simulink model "MenakaModel"  (R2022a)
settings: Solver=ode23tb  StartTime=0.0  StopTime=4  MaxStep=10/(60*24)  RelTol=1e-3
model workspace (MAT data in the model file):
  clima__A_c = 3295.16408265
  clima__A_f = 3100.53942116
  clima__G0 = [0.05; 0.00070738]
  clima__H = 7.9995824611
  clima__T0 = [287.15; 287.15; 287.15; 287.15]
  clima__T_ss = 280.150340169
  clima__alpha_c = 0.0100640347387
  clima__alpha_f = 0.0111385012129
  clima__alpha_i = 0.1
  clima__c_s = [1081 1081]
  clima__cd_c = 8736
  clima__d_c = 1.5
  clima__hour0 = 1
  clima__int_air_speed = 0.5
  clima__l_s = [0.1 0.1]
  clima__lam_s = [2.5 0.85]
  clima__minWindows = 0.299965865643
  clima__rhod_s = [2600 2500]
  clima__tau_c = 1
  crop__A_v = 2080
  crop__C = [0.01 0.001 0.01 0.01]
  crop__C_buf_max = 0.02
  crop__C_wv = 0.2
  crop__Chi_nutrients = [0.015625; 0.0104166666667; 0.00520833333333; 0.00208333333333; 0.00208333333333; 0.00104166666667; 0; 0]
  crop__N = [0; 0; 0; 0; 0; 0; 0; 0]
  crop__R = [0 0 0]
  crop__T_max_v = 40
  crop__T_max_v24 = 27
  crop__T_min_v = 6
  crop__T_min_v24 = 14
  crop__T_sum_end = 1035
  crop__T_v_start_fruit = 1100
  crop__Tsum = 0
  crop__Tv = 288
  crop__b_N_uptake = 0.5
  crop__c_fruit_g = 0.27
  crop__c_fruit_m = 2.3e-07
  crop__c_leaf_g = 0.28
  crop__c_leaf_m = 3.47e-07
  crop__c_stem_g = 0.3
  crop__c_stem_m = 1.47e-07
  crop__fraction_DM = 0.08
  crop__int_air_speed = 0.5
  crop__min_water_capacity = 0.1
  crop__plants_density = 2.1562
  crop__rg_fruit = 2e-07
  crop__rg_leaf = 9.5e-08
  crop__rg_stem = 7.4e-08
  crop__s_buforg_buf = -5000
  crop__s_max_T = 0.5793
  crop__s_max_T24 = 1.3904
  crop__s_min_T = -0.869
  crop__s_min_T24 = -1.1587
  heater__A_e = 0.0001
  heater__A_i = 0.008
  heater__T = 288
  heater__c = 5e-10
  heater__power = 60000000
  screen__Power = 100
  screen__Radthreshold = 900
  screen__beta = 2.23564167038e-14
  screen__gamma_max = 2.26308905438e-14
  screen__velocity = 0.333333333333
  subtrate__C_ws = 0.1
  subtrate__N = [0; 0; 0; 0; 0; 0; 0; 0]
  subtrate__Nmin_subs = 1e-09
  subtrate__Vmax_subs = 10
  subtrate__Vmin_subs = 0.01
  subtrate__sigma_max = 1
  subtrate__sigma_min = 1
  tomato__Cfruit0 = 0.001
  windows__AR = 19.9974923936
  windows__Power = 100
  windows__RadThreshold = 10
  windows__max_night = 10
  windows__tau = 600
undefined symbols (not defined in the file or in its folder): CO2_ppm_ext, Gain_control_Tv_mean, Gain_control_Tv_mean_superior, gain_max_night, GAIN_WIN, Hmax, Hstart, max_night, maxvelocity, RadTh_windows, Radthhold, shift_temp_heat, tau_win, tend_crop1, tend_crop2, tinit_crop1, tinit_crop2, Tmax, Tmax_mean, Tstart, Tven_max, Tven_start, WinAR
libraries: HORTISIM x26, simulink x6
(part 4 of 5)

== system MenakaModel/Control System/Control System Proportional (Ti) + Tmu Windows Relay/Windows Controler/Subsystem/Subsystem ==
  Tstart : Inport
  Ti : Inport  Port=2
  Tmax : Inport  Port=3
  Gain : Gain  Gain=100
  Subsystem2 : Subsystem
      settings: PortSchema="{\"entries\":[{\"content\":{\"sides\":[{\"content\":{\"connectorIds\":[\"In1\",\"In2\"]},\"type\":\"ConnectorPlacement.EquallySpacedRectSide\",\"uuid\":\"063c50bb-990a-4f1b-9201-b176301531ab\"},{\"content\":{\"connectorIds\":[\"Out1\"],\"side\":\"RIGHT\"},\"type\":\"ConnectorPlacement.EquallySpacedRectSide\",\"uuid\":\"3a0e99c4-d22b-4375-8de8-a1d36b289de2\"},{\"content\":{\"connectorIds\":[],\"side\":\"TOP\"},\"type\":\"ConnectorPlacement.EquallySpacedRectSide\",\"uuid\":\"03cb5fb9-820c-4863-975f-3967583da0d3\"},{\"content\":{\"connectorIds\":[\"In3\"],\"side\":\"BOTTOM\"},\"type\":\"ConnectorPlacement.EquallySpacedRectSide\",\"uuid\":\"69ae3c50-5771-48e7-9488-918c6831cfd5\"}]},\"type\":\"ConnectorPlacement.EquallySpacedConnector\",\"uuid\":\"dc439741-a5d5-4759-903e-5ad1ebb8fa8a\"}],\"packageUris\":[\"http://schema.mathworks.com/mf0/Connector/R2020b\"],\"version\":\"1.0\"}"
  y : Outport
  wires:
  Tstart/1 -> Subsystem2/2(" Min")
  Tmax/1 -> Subsystem2/1(Max)
  Ti/1 -> Subsystem2/3(T)
  Subsystem2/1(y) -> Gain/1
  Gain/1 -> y/1

== system MenakaModel/Control System/ON//OFF - constant setpoints/Subsystem1/Heating Controler/Subsystem ==
  T_i : Inport
  Q_h : Inport  Port=2
  T_e : Inport  Port=3
  Th : Inport  Port=4
  Constant : Constant  Value=A_i
  Constant1 : Constant  Value=c
  Constant2 : Constant  Value=A_e
  Product : Product
  Subsystem1 : Subsystem
  Subsystem2 : Subsystem
  Sum : Sum  Inputs=|-+-
  QV_h_i : Outport
  dT_h_dt : Outport  Port=2
  wires:
  T_i/1 -> Subsystem1/1(Ti)
  Constant/1 -> Subsystem1/2(A_h_exp)
  Th/1 -> Subsystem2/3(Th), Subsystem1/3(Th)
  T_e/1 -> Subsystem2/1(Te)
  Subsystem1/1(QV_h_i) -> QV_h_i/1, Sum/1
  Subsystem2/1(QV_h_e) -> Sum/3
  Q_h/1 -> Sum/2
  Sum/1 -> Product/1
  Constant1/1 -> Product/2
  Product/1 -> dT_h_dt/1
  Constant2/1 -> Subsystem2/2(A_h_exp)

== system MenakaModel/Control System/ON//OFF - constant setpoints/Subsystem1/Subsystem2/If Action Subsystem ==
  Action Port : ActionPort  ActionPortLabel=if(u2 > u1)
  Constant : Constant  Value=0
  Out1 : Outport
  wires:
  Constant/1 -> Out1/1

== system MenakaModel/Control System/ON//OFF - constant setpoints/Subsystem1/Subsystem2/If Action Subsystem1 ==
  Action Port : ActionPort  ActionPortLabel=elseif(u2 < u3)
  Constant : Constant
  Out1 : Outport
  wires:
  Constant/1 -> Out1/1

== system MenakaModel/Control System/ON//OFF - constant setpoints/Subsystem1/Subsystem2/If Action Subsystem2 ==
  In1 : Inport
  Action Port : ActionPort  ActionPortLabel=else
  Out1 : Outport
  wires:
  In1/1 -> Out1/1

== system MenakaModel/Control System/ON//OFF - constant setpoints/Subsystem1/Windows Controler/Subsystem ==
  Tstart : Inport
  Ti : Inport  Port=2
  Tmax : Inport  Port=3
  HRInt : Inport  Port=4
  HRStart : Inport  Port=5
  HRMax : Inport  Port=6
  Rad : Inport  Port=7
  max_night : Inport  Port=8
  Constant : Constant  Value=RadThreshold
  Constant1 : Constant  Value=0
  Saturation Dynamic : simulink/Discontinuities/Saturation Dynamic  OutMin=[]  OutMax=[]  OutDataTypeStr=Inherit: Same as second input  OutDataType=fixdt(1, 16)  OutScaling=2^-10  DoSatur=off
  "Selection " : MATLAB Function  TreatAsAtomicUnit=on
  Temp : Saturate  UpperLimit=100  LowerLimit=0
  Temp1 : Saturate  UpperLimit=100  LowerLimit=0
  Ventilation by Hight Humidity : MATLAB Function  TreatAsAtomicUnit=on
  Ventilation by Hight Temperature1 : MATLAB Function  TreatAsAtomicUnit=on
  y : Outport
  wires:
  Ti/1 -> Ventilation by Hight Temperature1/2(Ti)
  Rad/1 -> "Selection "/1(Rad)
  Tstart/1 -> Ventilation by Hight Temperature1/1(Tstart)
  HRMax/1 -> Ventilation by Hight Humidity/3(HRMax)
  Tmax/1 -> Ventilation by Hight Temperature1/3(Tmax)
  "Selection "/1(y) -> y/1
  Ventilation by Hight Humidity/1(y) -> Saturation Dynamic/2
  HRStart/1 -> Ventilation by Hight Humidity/2(HRStart)
  Ventilation by Hight Temperature1/1(y) -> Temp/1
  HRInt/1 -> Ventilation by Hight Humidity/1(HRInt)
  Temp/1 -> "Selection "/2(Temperature)
  Constant/1 -> "Selection "/4(Rad_threshold)
  Constant1/1 -> Saturation Dynamic/3
  max_night/1 -> Saturation Dynamic/1
  Saturation Dynamic/1 -> Temp1/1
  Temp1/1 -> "Selection "/3(Humidity)

== system MenakaModel/Control System/PID - const st - Ti mesure - Dynamics ST/Subsystem1/Heating Controler/Subsystem ==
  T_i : Inport
  Q_h : Inport  Port=2
  T_e : Inport  Port=3
  Th : Inport  Port=4
  Constant : Constant  Value=A_i
  Constant1 : Constant  Value=c
  Constant2 : Constant  Value=A_e
  Product : Product
  Subsystem1 : Subsystem
  Subsystem2 : Subsystem
  Sum : Sum  Inputs=|-+-
  QV_h_i : Outport
  dT_h_dt : Outport  Port=2
  wires:
  T_i/1 -> Subsystem1/1(Ti)
  Constant/1 -> Subsystem1/2(A_h_exp)
  Th/1 -> Subsystem2/3(Th), Subsystem1/3(Th)
  T_e/1 -> Subsystem2/1(Te)
  Subsystem1/1(QV_h_i) -> QV_h_i/1, Sum/1
  Subsystem2/1(QV_h_e) -> Sum/3
  Q_h/1 -> Sum/2
  Sum/1 -> Product/1
  Constant1/1 -> Product/2
  Product/1 -> dT_h_dt/1
  Constant2/1 -> Subsystem2/2(A_h_exp)

== system MenakaModel/Control System/PID - const st - Ti mesure - Dynamics ST/Subsystem1/Subsystem2/PI ==
  Max : Inport
  " Min" : Inport  Port=2
  T : Inport  Port=3
  In Bus Element : Inport  Port=4  PortName=IC  Element=Temp.Tair
  Gain : Gain
  Gain1 : Gain  Gain=0.5
  Gain2 : Gain  Gain=0.1
  Integrator : Integrator
  Minus : Sum  Inputs=+-
  Saturation : Saturate  UpperLimit=1  LowerLimit=0
  Sum : Sum  Inputs=|++
  Sum1 : Sum  Inputs=|++
  y : Outport
  wires:
  In Bus Element/1 -> Minus/2
  Saturation/1 -> y/1
  " Min"/1 -> Minus/1
  Minus/1 -> Integrator/1, Gain/1
  Max/1 -> Gain1/1
  Gain1/1 -> Sum/1
  Integrator/1 -> Gain2/1
  Sum1/1 -> Saturation/1
  Gain/1 -> Sum1/1
  Gain2/1 -> Sum1/2

== system MenakaModel/Control System/PID - const st - Ti mesure - Dynamics ST/Subsystem1/Subsystem2/Subsystem2 ==
  Max : Inport
  " Min" : Inport  Port=2
  T : Inport  Port=3
  In Bus Element : Inport  Port=4  PortName=IC  Element=Temp.Tair
  Gain : Gain
  Gain1 : Gain  Gain=0.5
  Minus : Sum  Inputs=+-
  Saturation : Saturate  UpperLimit=1  LowerLimit=0
  Sum : Sum  Inputs=|++
  y : Outport
  wires:
  Max/1 -> Gain1/1
  Gain/1 -> Saturation/1
  Minus/1 -> Gain/1
  Saturation/1 -> y/1
  Gain1/1 -> Sum/1
  " Min"/1 -> Minus/1
  In Bus Element/1 -> Minus/2

== system MenakaModel/Control System/PID - const st - Ti mesure - Dynamics ST/Subsystem1/Windows Controler/Subsystem ==
  Tstart : Inport
  Ti : Inport  Port=2
  Tmax : Inport  Port=3
  HRInt : Inport  Port=4
  HRStart : Inport  Port=5
  HRMax : Inport  Port=6
  Rad : Inport  Port=7
  max_night : Inport  Port=8
  Constant : Constant  Value=RadThreshold
  Constant1 : Constant  Value=0
  Saturation Dynamic : simulink/Discontinuities/Saturation Dynamic  OutMin=[]  OutMax=[]  OutDataTypeStr=Inherit: Same as second input  OutDataType=fixdt(1, 16)  OutScaling=2^-10  DoSatur=off
  "Selection " : MATLAB Function  TreatAsAtomicUnit=on
  Temp : Saturate  UpperLimit=100  LowerLimit=0
  Temp1 : Saturate  UpperLimit=100  LowerLimit=0
  Ventilation by Hight Humidity : MATLAB Function  TreatAsAtomicUnit=on
  Ventilation by Hight Temperature1 : MATLAB Function  TreatAsAtomicUnit=on
  y : Outport
  wires:
  Ti/1 -> Ventilation by Hight Temperature1/2(Ti)
  Rad/1 -> "Selection "/1(Rad)
  Tstart/1 -> Ventilation by Hight Temperature1/1(Tstart)
  HRMax/1 -> Ventilation by Hight Humidity/3(HRMax)
  Tmax/1 -> Ventilation by Hight Temperature1/3(Tmax)
  "Selection "/1(y) -> y/1
  Ventilation by Hight Humidity/1(y) -> Saturation Dynamic/2
  HRStart/1 -> Ventilation by Hight Humidity/2(HRStart)
  Ventilation by Hight Temperature1/1(y) -> Temp/1
  HRInt/1 -> Ventilation by Hight Humidity/1(HRInt)
  Temp/1 -> "Selection "/2(Temperature)
  Constant/1 -> "Selection "/4(Rad_threshold)
  Constant1/1 -> Saturation Dynamic/3
  max_night/1 -> Saturation Dynamic/1
  Saturation Dynamic/1 -> Temp1/1
  Temp1/1 -> "Selection "/3(Humidity)

== system MenakaModel/Control System/PID - constant setpoints/Subsystem1/Heating Controler/Subsystem ==
  T_i : Inport
  Q_h : Inport  Port=2
  T_e : Inport  Port=3
  Th : Inport  Port=4
  Constant : Constant  Value=A_i
  Constant1 : Constant  Value=c
  Constant2 : Constant  Value=A_e
  Product : Product
  Subsystem1 : Subsystem
  Subsystem2 : Subsystem
  Sum : Sum  Inputs=|-+-
  QV_h_i : Outport
  dT_h_dt : Outport  Port=2
  wires:
  T_i/1 -> Subsystem1/1(Ti)
  Constant/1 -> Subsystem1/2(A_h_exp)
  Th/1 -> Subsystem2/3(Th), Subsystem1/3(Th)
  T_e/1 -> Subsystem2/1(Te)
  Subsystem1/1(QV_h_i) -> QV_h_i/1, Sum/1
  Subsystem2/1(QV_h_e) -> Sum/3
  Q_h/1 -> Sum/2
  Sum/1 -> Product/1
  Constant1/1 -> Product/2
  Product/1 -> dT_h_dt/1
  Constant2/1 -> Subsystem2/2(A_h_exp)

== system MenakaModel/Control System/PID - constant setpoints/Subsystem1/Windows Controler/Subsystem ==
  Tstart : Inport
  Ti : Inport  Port=2
  Tmax : Inport  Port=3
  HRInt : Inport  Port=4
  HRStart : Inport  Port=5
  HRMax : Inport  Port=6
  Rad : Inport  Port=7
  max_night : Inport  Port=8
  Constant : Constant  Value=RadThreshold
  Constant1 : Constant  Value=0
  Saturation Dynamic : simulink/Discontinuities/Saturation Dynamic  OutMin=[]  OutMax=[]  OutDataTypeStr=Inherit: Same as second input  OutDataType=fixdt(1, 16)  OutScaling=2^-10  DoSatur=off
  "Selection " : MATLAB Function  TreatAsAtomicUnit=on
  Temp : Saturate  UpperLimit=100  LowerLimit=0
  Temp1 : Saturate  UpperLimit=100  LowerLimit=0
  Ventilation by Hight Humidity : MATLAB Function  TreatAsAtomicUnit=on
  Ventilation by Hight Temperature1 : MATLAB Function  TreatAsAtomicUnit=on
  y : Outport
  wires:
  Ti/1 -> Ventilation by Hight Temperature1/2(Ti)
  Rad/1 -> "Selection "/1(Rad)
  Tstart/1 -> Ventilation by Hight Temperature1/1(Tstart)
  HRMax/1 -> Ventilation by Hight Humidity/3(HRMax)
  Tmax/1 -> Ventilation by Hight Temperature1/3(Tmax)
  "Selection "/1(y) -> y/1
  Ventilation by Hight Humidity/1(y) -> Saturation Dynamic/2
  HRStart/1 -> Ventilation by Hight Humidity/2(HRStart)
  Ventilation by Hight Temperature1/1(y) -> Temp/1
  HRInt/1 -> Ventilation by Hight Humidity/1(HRInt)
  Temp/1 -> "Selection "/2(Temperature)
  Constant/1 -> "Selection "/4(Rad_threshold)
  Constant1/1 -> Saturation Dynamic/3
  max_night/1 -> Saturation Dynamic/1
  Saturation Dynamic/1 -> Temp1/1
  Temp1/1 -> "Selection "/3(Humidity)

== system MenakaModel/Control System/PID - constant setpoints - Ti measure/Subsystem1/Heating Controler/Subsystem ==
  T_i : Inport
  Q_h : Inport  Port=2
  T_e : Inport  Port=3
  Th : Inport  Port=4
  Constant : Constant  Value=A_i
  Constant1 : Constant  Value=c
  Constant2 : Constant  Value=A_e
  Product : Product
  Subsystem1 : Subsystem
  Subsystem2 : Subsystem
  Sum : Sum  Inputs=|-+-
  QV_h_i : Outport
  dT_h_dt : Outport  Port=2
  wires:
  T_i/1 -> Subsystem1/1(Ti)
  Constant/1 -> Subsystem1/2(A_h_exp)
  Th/1 -> Subsystem2/3(Th), Subsystem1/3(Th)
  T_e/1 -> Subsystem2/1(Te)
  Subsystem1/1(QV_h_i) -> QV_h_i/1, Sum/1
  Subsystem2/1(QV_h_e) -> Sum/3
  Q_h/1 -> Sum/2
  Sum/1 -> Product/1
  Constant1/1 -> Product/2
  Product/1 -> dT_h_dt/1
  Constant2/1 -> Subsystem2/2(A_h_exp)

== system MenakaModel/Control System/PID - constant setpoints - Ti measure/Subsystem1/Subsystem2/PI ==
  Max : Inport
  " Min" : Inport  Port=2
  T : Inport  Port=3
  In Bus Element : Inport  Port=4  PortName=IC  Element=Temp.Tair
  Gain : Gain
  Gain1 : Gain  Gain=0.5
  Gain2 : Gain  Gain=0.1
  Integrator : Integrator
  Minus : Sum  Inputs=+-
  Saturation : Saturate  UpperLimit=1  LowerLimit=0
  Sum : Sum  Inputs=|++
  Sum1 : Sum  Inputs=|++
  y : Outport
  wires:
  In Bus Element/1 -> Minus/2
  Saturation/1 -> y/1
  " Min"/1 -> Minus/1
  Minus/1 -> Integrator/1, Gain/1
  Max/1 -> Gain1/1
  Gain1/1 -> Sum/1
  Integrator/1 -> Gain2/1
  Sum1/1 -> Saturation/1
  Gain/1 -> Sum1/1
  Gain2/1 -> Sum1/2

== system MenakaModel/Control System/PID - constant setpoints - Ti measure/Subsystem1/Subsystem2/Subsystem2 ==
  Max : Inport
  " Min" : Inport  Port=2
  T : Inport  Port=3
  In Bus Element : Inport  Port=4  PortName=IC  Element=Temp.Tair
  Gain : Gain
  Gain1 : Gain  Gain=0.5
  Minus : Sum  Inputs=+-
  Saturation : Saturate  UpperLimit=1  LowerLimit=0
  Sum : Sum  Inputs=|++
  y : Outport
  wires:
  Max/1 -> Gain1/1
  Gain/1 -> Saturation/1
  Minus/1 -> Gain/1
  Saturation/1 -> y/1
  Gain1/1 -> Sum/1
  " Min"/1 -> Minus/1
  In Bus Element/1 -> Minus/2

== system MenakaModel/Control System/PID - constant setpoints - Ti measure/Subsystem1/Windows Controler/Subsystem ==
  Tstart : Inport
  Ti : Inport  Port=2
  Tmax : Inport  Port=3
  HRInt : Inport  Port=4
  HRStart : Inport  Port=5
  HRMax : Inport  Port=6
  Rad : Inport  Port=7
  max_night : Inport  Port=8
  Constant : Constant  Value=RadThreshold
  Constant1 : Constant  Value=0
  Saturation Dynamic : simulink/Discontinuities/Saturation Dynamic  OutMin=[]  OutMax=[]  OutDataTypeStr=Inherit: Same as second input  OutDataType=fixdt(1, 16)  OutScaling=2^-10  DoSatur=off
  "Selection " : MATLAB Function  TreatAsAtomicUnit=on
  Temp : Saturate  UpperLimit=100  LowerLimit=0
  Temp1 : Saturate  UpperLimit=100  LowerLimit=0
  Ventilation by Hight Humidity : MATLAB Function  TreatAsAtomicUnit=on
  Ventilation by Hight Temperature1 : MATLAB Function  TreatAsAtomicUnit=on
  y : Outport
  wires:
  Ti/1 -> Ventilation by Hight Temperature1/2(Ti)
  Rad/1 -> "Selection "/1(Rad)
  Tstart/1 -> Ventilation by Hight Temperature1/1(Tstart)
  HRMax/1 -> Ventilation by Hight Humidity/3(HRMax)
  Tmax/1 -> Ventilation by Hight Temperature1/3(Tmax)
  "Selection "/1(y) -> y/1
  Ventilation by Hight Humidity/1(y) -> Saturation Dynamic/2
  HRStart/1 -> Ventilation by Hight Humidity/2(HRStart)
  Ventilation by Hight Temperature1/1(y) -> Temp/1
  HRInt/1 -> Ventilation by Hight Humidity/1(HRInt)
  Temp/1 -> "Selection "/2(Temperature)
  Constant/1 -> "Selection "/4(Rad_threshold)
  Constant1/1 -> Saturation Dynamic/3
  max_night/1 -> Saturation Dynamic/1
  Saturation Dynamic/1 -> Temp1/1
  Temp1/1 -> "Selection "/3(Humidity)

== system MenakaModel/Control System/PID-set-points/Subsystem1/Heating Controler/Subsystem ==
  T_i : Inport
  Q_h : Inport  Port=2
  T_e : Inport  Port=3
  Th : Inport  Port=4
  Constant : Constant  Value=A_i
  Constant1 : Constant  Value=c
  Constant2 : Constant  Value=A_e
  Product : Product
  Subsystem1 : Subsystem
  Subsystem2 : Subsystem
  Sum : Sum  Inputs=|-+-
  QV_h_i : Outport
  dT_h_dt : Outport  Port=2
  wires:
  T_i/1 -> Subsystem1/1(Ti)
  Constant/1 -> Subsystem1/2(A_h_exp)
  Th/1 -> Subsystem2/3(Th), Subsystem1/3(Th)
  T_e/1 -> Subsystem2/1(Te)
  Subsystem1/1(QV_h_i) -> QV_h_i/1, Sum/1
  Subsystem2/1(QV_h_e) -> Sum/3
  Q_h/1 -> Sum/2
  Sum/1 -> Product/1
  Constant1/1 -> Product/2
  Product/1 -> dT_h_dt/1
  Constant2/1 -> Subsystem2/2(A_h_exp)

== system MenakaModel/Control System/PID-set-points/Subsystem1/Windows Controler/Subsystem ==
  Tstart : Inport
  Ti : Inport  Port=2
  Tmax : Inport  Port=3
  HRInt : Inport  Port=4
  HRStart : Inport  Port=5
  HRMax : Inport  Port=6
  Rad : Inport  Port=7
  max_night : Inport  Port=8
  Constant : Constant  Value=RadThreshold
  Constant1 : Constant  Value=0
  Saturation Dynamic : simulink/Discontinuities/Saturation Dynamic  OutMin=[]  OutMax=[]  OutDataTypeStr=Inherit: Same as second input  OutDataType=fixdt(1, 16)  OutScaling=2^-10  DoSatur=off
  "Selection " : MATLAB Function  TreatAsAtomicUnit=on
  Temp : Saturate  UpperLimit=100  LowerLimit=0
  Temp1 : Saturate  UpperLimit=100  LowerLimit=0
  Ventilation by Hight Humidity : MATLAB Function  TreatAsAtomicUnit=on
  Ventilation by Hight Temperature1 : MATLAB Function  TreatAsAtomicUnit=on
  y : Outport
  wires:
  Ti/1 -> Ventilation by Hight Temperature1/2(Ti)
  Rad/1 -> "Selection "/1(Rad)
  Tstart/1 -> Ventilation by Hight Temperature1/1(Tstart)
  HRMax/1 -> Ventilation by Hight Humidity/3(HRMax)
  Tmax/1 -> Ventilation by Hight Temperature1/3(Tmax)
  "Selection "/1(y) -> y/1
  Ventilation by Hight Humidity/1(y) -> Saturation Dynamic/2
  HRStart/1 -> Ventilation by Hight Humidity/2(HRStart)
  Ventilation by Hight Temperature1/1(y) -> Temp/1
  HRInt/1 -> Ventilation by Hight Humidity/1(HRInt)
  Temp/1 -> "Selection "/2(Temperature)
  Constant/1 -> "Selection "/4(Rad_threshold)
  Constant1/1 -> Saturation Dynamic/3
  max_night/1 -> Saturation Dynamic/1
  Saturation Dynamic/1 -> Temp1/1
  Temp1/1 -> "Selection "/3(Humidity)

== system MenakaModel/Control System/Setpoints Control - ON//OFF/Subsystem1/Heating Controler/Subsystem ==
  T_i : Inport
  Q_h : Inport  Port=2
  T_e : Inport  Port=3
  Th : Inport  Port=4
  Constant : Constant  Value=A_i
  Constant1 : Constant  Value=c
  Constant2 : Constant  Value=A_e
  Product : Product
  Subsystem1 : Subsystem
  Subsystem2 : Subsystem
  Sum : Sum  Inputs=|-+-
  QV_h_i : Outport
  dT_h_dt : Outport  Port=2
  wires:
  T_i/1 -> Subsystem1/1(Ti)
  Constant/1 -> Subsystem1/2(A_h_exp)
  Th/1 -> Subsystem2/3(Th), Subsystem1/3(Th)
  T_e/1 -> Subsystem2/1(Te)
  Subsystem1/1(QV_h_i) -> QV_h_i/1, Sum/1
  Subsystem2/1(QV_h_e) -> Sum/3
  Q_h/1 -> Sum/2
  Sum/1 -> Product/1
  Constant1/1 -> Product/2
  Product/1 -> dT_h_dt/1
  Constant2/1 -> Subsystem2/2(A_h_exp)

== system MenakaModel/Control System/Setpoints Control - ON//OFF/Subsystem1/Subsystem2/If Action Subsystem ==
  Action Port : ActionPort  ActionPortLabel=if(u2 > u1)
  Constant : Constant  Value=0
  Out1 : Outport
  wires:
  Constant/1 -> Out1/1

== system MenakaModel/Control System/Setpoints Control - ON//OFF/Subsystem1/Subsystem2/If Action Subsystem1 ==
  Action Port : ActionPort  ActionPortLabel=elseif(u2 < u3)
  Constant : Constant
  Out1 : Outport
  wires:
  Constant/1 -> Out1/1

== system MenakaModel/Control System/Setpoints Control - ON//OFF/Subsystem1/Subsystem2/If Action Subsystem2 ==
  In1 : Inport
  Action Port : ActionPort  ActionPortLabel=else
  Out1 : Outport
  wires:
  In1/1 -> Out1/1

== system MenakaModel/Control System/Setpoints Control - ON//OFF/Subsystem1/Windows Controler/Subsystem ==
  Tstart : Inport
  Ti : Inport  Port=2
  Tmax : Inport  Port=3
  HRInt : Inport  Port=4
  HRStart : Inport  Port=5
  HRMax : Inport  Port=6
  Rad : Inport  Port=7
  max_night : Inport  Port=8
  Constant : Constant  Value=RadThreshold
  Constant1 : Constant  Value=0
  Saturation Dynamic : simulink/Discontinuities/Saturation Dynamic  OutMin=[]  OutMax=[]  OutDataTypeStr=Inherit: Same as second input  OutDataType=fixdt(1, 16)  OutScaling=2^-10  DoSatur=off
  "Selection " : MATLAB Function  TreatAsAtomicUnit=on
  Temp : Saturate  UpperLimit=100  LowerLimit=0
  Temp1 : Saturate  UpperLimit=100  LowerLimit=0
  Ventilation by Hight Humidity : MATLAB Function  TreatAsAtomicUnit=on
  Ventilation by Hight Temperature1 : MATLAB Function  TreatAsAtomicUnit=on
  y : Outport
  wires:
  Ti/1 -> Ventilation by Hight Temperature1/2(Ti)
  Rad/1 -> "Selection "/1(Rad)
  Tstart/1 -> Ventilation by Hight Temperature1/1(Tstart)
  HRMax/1 -> Ventilation by Hight Humidity/3(HRMax)
  Tmax/1 -> Ventilation by Hight Temperature1/3(Tmax)
  "Selection "/1(y) -> y/1
  Ventilation by Hight Humidity/1(y) -> Saturation Dynamic/2
  HRStart/1 -> Ventilation by Hight Humidity/2(HRStart)
  Ventilation by Hight Temperature1/1(y) -> Temp/1
  HRInt/1 -> Ventilation by Hight Humidity/1(HRInt)
  Temp/1 -> "Selection "/2(Temperature)
  Constant/1 -> "Selection "/4(Rad_threshold)
  Constant1/1 -> Saturation Dynamic/3
  max_night/1 -> Saturation Dynamic/1
  Saturation Dynamic/1 -> Temp1/1
  Temp1/1 -> "Selection "/3(Humidity)

== system MenakaModel/Control System/Control System Proportional (Ti) + Tmu /Heating Controler/Subsystem/Subsystem1/Subsystem ==
  Ti : Inport
  Th : Inport  Port=2
  " nu kinematic viscosity [m^2/s]" : Constant  Value=15.1e-6
  Abs : Abs  SaturateOnIntegerOverflow=off
  Constant : Constant  Value=3
  Divide : Product  Inputs=*/
  Divide1 : Product  Inputs=*/
  Minus : Sum  Inputs=+-
  Power : Math  Operator=pow
  Product : Product
  Product1 : Product
  Square : Math  Operator=square
  d_h : Constant  Value=1.5
  g acceleration due to gravity [m/s^2] : Constant  Value=9.81
  Gr : Outport
  dT : Outport  Port=2
  wires:
  g acceleration due to gravity [m/s^2]/1 -> Product/1
  Abs/1 -> Divide/1
  Divide1/1 -> Product1/1
  Divide/1 -> Product1/2
  Product1/1 -> Gr/1
  Square/1 -> Divide1/2
  Product/1 -> Divide1/1
  Constant/1 -> Power/2
  Th/1 -> Minus/1
  " nu kinematic viscosity [m^2/s]"/1 -> Square/1
  Minus/1 -> dT/1, Abs/1
  d_h/1 -> Power/1
  Power/1 -> Product/2
  Ti/1 -> Divide/2, Minus/2

== system MenakaModel/Control System/Control System Proportional (Ti) + Tmu /Heating Controler/Subsystem/Subsystem2/Subsystem ==
  Ti : Inport
  Th : Inport  Port=2
  " nu kinematic viscosity [m^2/s]" : Constant  Value=15.1e-6
  Abs : Abs  SaturateOnIntegerOverflow=off
  Constant : Constant  Value=3
  Divide : Product  Inputs=*/
  Divide1 : Product  Inputs=*/
  Minus : Sum  Inputs=+-
  Power : Math  Operator=pow
  Product : Product
  Product1 : Product
  Square : Math  Operator=square
  d_h : Constant  Value=1.5
  g acceleration due to gravity [m/s^2] : Constant  Value=9.81
  Gr : Outport
  dT : Outport  Port=2
  wires:
  g acceleration due to gravity [m/s^2]/1 -> Product/1
  Abs/1 -> Divide/1
  Divide1/1 -> Product1/1
  Divide/1 -> Product1/2
  Product1/1 -> Gr/1
  Square/1 -> Divide1/2
  Product/1 -> Divide1/1
  Constant/1 -> Power/2
  Th/1 -> Minus/1
  " nu kinematic viscosity [m^2/s]"/1 -> Square/1
  Minus/1 -> dT/1, Abs/1
  d_h/1 -> Power/1
  Power/1 -> Product/2
  Ti/1 -> Divide/2, Minus/2

== system MenakaModel/Control System/Control System Proportional (Ti) + Tmu Windows Relay/Heating Controler/Subsystem/Subsystem1/Subsystem ==
  Ti : Inport
  Th : Inport  Port=2
  " nu kinematic viscosity [m^2/s]" : Constant  Value=15.1e-6
  Abs : Abs  SaturateOnIntegerOverflow=off
  Constant : Constant  Value=3
  Divide : Product  Inputs=*/
  Divide1 : Product  Inputs=*/
  Minus : Sum  Inputs=+-
  Power : Math  Operator=pow
  Product : Product
  Product1 : Product
  Square : Math  Operator=square
  d_h : Constant  Value=1.5
  g acceleration due to gravity [m/s^2] : Constant  Value=9.81
  Gr : Outport
  dT : Outport  Port=2
  wires:
  g acceleration due to gravity [m/s^2]/1 -> Product/1
  Abs/1 -> Divide/1
  Divide1/1 -> Product1/1
  Divide/1 -> Product1/2
  Product1/1 -> Gr/1
  Square/1 -> Divide1/2
  Product/1 -> Divide1/1
  Constant/1 -> Power/2
  Th/1 -> Minus/1
  " nu kinematic viscosity [m^2/s]"/1 -> Square/1
  Minus/1 -> dT/1, Abs/1
  d_h/1 -> Power/1
  Power/1 -> Product/2
  Ti/1 -> Divide/2, Minus/2

== system MenakaModel/Control System/Control System Proportional (Ti) + Tmu Windows Relay/Heating Controler/Subsystem/Subsystem2/Subsystem ==
  Ti : Inport
  Th : Inport  Port=2
  " nu kinematic viscosity [m^2/s]" : Constant  Value=15.1e-6
  Abs : Abs  SaturateOnIntegerOverflow=off
  Constant : Constant  Value=3
  Divide : Product  Inputs=*/
  Divide1 : Product  Inputs=*/
  Minus : Sum  Inputs=+-
  Power : Math  Operator=pow
  Product : Product
  Product1 : Product
  Square : Math  Operator=square
  d_h : Constant  Value=1.5
  g acceleration due to gravity [m/s^2] : Constant  Value=9.81
  Gr : Outport
  dT : Outport  Port=2
  wires:
  g acceleration due to gravity [m/s^2]/1 -> Product/1
  Abs/1 -> Divide/1
  Divide1/1 -> Product1/1
  Divide/1 -> Product1/2
  Product1/1 -> Gr/1
  Square/1 -> Divide1/2
  Product/1 -> Divide1/1
  Constant/1 -> Power/2
  Th/1 -> Minus/1
  " nu kinematic viscosity [m^2/s]"/1 -> Square/1
  Minus/1 -> dT/1, Abs/1
  d_h/1 -> Power/1
  Power/1 -> Product/2
  Ti/1 -> Divide/2, Minus/2

== system MenakaModel/Control System/Control System Proportional (Ti) + Tmu Windows Relay/Screen Controler/Subsystem/If Action Subsystem1/Theta  ==
  In1 : Inport
  Constant1 : Constant  Value=0.5
  Gain : Gain  Gain=0.5
  Sign : Signum  ZeroCross=off
  Sum : Sum  Inputs=|++
  Out1 : Outport
  wires:
  Sign/1 -> Gain/1
  Sum/1 -> Out1/1
  Gain/1 -> Sum/1
  In1/1 -> Sign/1
  Constant1/1 -> Sum/2

== system MenakaModel/Control System/Control System Proportional (Ti) + Tmu Windows Relay/Windows Controler/Subsystem/Subsystem/Subsystem2 ==
  Max : Inport
  " Min" : Inport  Port=2
  T : Inport  Port=3
  If : If  NumInputs=3  IfExpression=u2 > u1  ElseIfExpressions=u2 < u3
  If Action Subsystem : Subsystem  TreatAsAtomicUnit=on
  If Action Subsystem1 : Subsystem  TreatAsAtomicUnit=on
  If Action Subsystem2 : Subsystem  TreatAsAtomicUnit=on
  Memory : Memory  InitialCondition=2/(60*24)  InheritSampleTime=on
  Merge : Merge  Inputs=3
  y : Outport
  wires:
  " Min"/1 -> If/3
  If Action Subsystem/1(Out1) -> Merge/1
  Max/1 -> If/1
  If/1 -> If Action Subsystem/Action
  Merge/1 -> y/1, Memory/1
  Memory/1 -> If Action Subsystem2/1(In1)
  If/2 -> If Action Subsystem1/Action
  T/1 -> If/2
  If Action Subsystem1/1(Out1) -> Merge/2
  If/3 -> If Action Subsystem2/Action
  If Action Subsystem2/1(Out1) -> Merge/3

== system MenakaModel/Control System/ON//OFF - constant setpoints/Subsystem1/Heating Controler/Subsystem/Subsystem1 ==
  Ti : Inport
  A_h_exp : Inport  Port=2
  Th : Inport  Port=3
  Divide2 : Product  Inputs=****/
  Subsystem : Subsystem
  d_h1 : Constant  Value=1.5
  lambda thermal conductivity of air [W/m/K] : Constant  Value=0.025
  QV_h_i : Outport
  wires:
  Divide2/1 -> QV_h_i/1
  Subsystem/2(dT) -> Divide2/4
  Subsystem/1(Gr) -> Divide2/2
  d_h1/1 -> Divide2/5
  A_h_exp/1 -> Divide2/3
  lambda thermal conductivity of air [W/m/K]/1 -> Divide2/1
  Th/1 -> Subsystem/2(Th)
  Ti/1 -> Subsystem/1(Ti)

== system MenakaModel/Control System/ON//OFF - constant setpoints/Subsystem1/Heating Controler/Subsystem/Subsystem2 ==
  Te : Inport
  A_h_exp : Inport  Port=2
  Th : Inport  Port=3
  Divide2 : Product  Inputs=****/
  Subsystem : Subsystem
  d_h1 : Constant  Value=1.5
  lambda thermal conductivity of air [W/m/K] : Constant  Value=0.025
  QV_h_e : Outport
  wires:
  Divide2/1 -> QV_h_e/1
  Subsystem/2(dT) -> Divide2/4
  Subsystem/1(Gr) -> Divide2/2
  d_h1/1 -> Divide2/5
  A_h_exp/1 -> Divide2/3
  lambda thermal conductivity of air [W/m/K]/1 -> Divide2/1
  Th/1 -> Subsystem/2(Th)
  Te/1 -> Subsystem/1(Ti)

== system MenakaModel/Control System/PID - const st - Ti mesure - Dynamics ST/Subsystem1/Heating Controler/Subsystem/Subsystem1 ==
  Ti : Inport
  A_h_exp : Inport  Port=2
  Th : Inport  Port=3
  Divide2 : Product  Inputs=****/
  Subsystem : Subsystem
  d_h1 : Constant  Value=1.5
  lambda thermal conductivity of air [W/m/K] : Constant  Value=0.025
  QV_h_i : Outport
  wires:
  Divide2/1 -> QV_h_i/1
  Subsystem/2(dT) -> Divide2/4
  Subsystem/1(Gr) -> Divide2/2
  d_h1/1 -> Divide2/5
  A_h_exp/1 -> Divide2/3
  lambda thermal conductivity of air [W/m/K]/1 -> Divide2/1
  Th/1 -> Subsystem/2(Th)
  Ti/1 -> Subsystem/1(Ti)

== system MenakaModel/Control System/PID - const st - Ti mesure - Dynamics ST/Subsystem1/Heating Controler/Subsystem/Subsystem2 ==
  Te : Inport
  A_h_exp : Inport  Port=2
  Th : Inport  Port=3
  Divide2 : Product  Inputs=****/
  Subsystem : Subsystem
  d_h1 : Constant  Value=1.5
  lambda thermal conductivity of air [W/m/K] : Constant  Value=0.025
  QV_h_e : Outport
  wires:
  Divide2/1 -> QV_h_e/1
  Subsystem/2(dT) -> Divide2/4
  Subsystem/1(Gr) -> Divide2/2
  d_h1/1 -> Divide2/5
  A_h_exp/1 -> Divide2/3
  lambda thermal conductivity of air [W/m/K]/1 -> Divide2/1
  Th/1 -> Subsystem/2(Th)
  Te/1 -> Subsystem/1(Ti)

== system MenakaModel/Control System/PID - constant setpoints/Subsystem1/Heating Controler/Subsystem/Subsystem1 ==
  Ti : Inport
  A_h_exp : Inport  Port=2
  Th : Inport  Port=3
  Divide2 : Product  Inputs=****/
  Subsystem : Subsystem
  d_h1 : Constant  Value=1.5
  lambda thermal conductivity of air [W/m/K] : Constant  Value=0.025
  QV_h_i : Outport
  wires:
  Divide2/1 -> QV_h_i/1
  Subsystem/2(dT) -> Divide2/4
  Subsystem/1(Gr) -> Divide2/2
  d_h1/1 -> Divide2/5
  A_h_exp/1 -> Divide2/3
  lambda thermal conductivity of air [W/m/K]/1 -> Divide2/1
  Th/1 -> Subsystem/2(Th)
  Ti/1 -> Subsystem/1(Ti)

== system MenakaModel/Control System/PID - constant setpoints/Subsystem1/Heating Controler/Subsystem/Subsystem2 ==
  Te : Inport
  A_h_exp : Inport  Port=2
  Th : Inport  Port=3
  Divide2 : Product  Inputs=****/
  Subsystem : Subsystem
  d_h1 : Constant  Value=1.5
  lambda thermal conductivity of air [W/m/K] : Constant  Value=0.025
  QV_h_e : Outport
  wires:
  Divide2/1 -> QV_h_e/1
  Subsystem/2(dT) -> Divide2/4
  Subsystem/1(Gr) -> Divide2/2
  d_h1/1 -> Divide2/5
  A_h_exp/1 -> Divide2/3
  lambda thermal conductivity of air [W/m/K]/1 -> Divide2/1
  Th/1 -> Subsystem/2(Th)
  Te/1 -> Subsystem/1(Ti)

== system MenakaModel/Control System/PID - constant setpoints - Ti measure/Subsystem1/Heating Controler/Subsystem/Subsystem1 ==
  Ti : Inport
  A_h_exp : Inport  Port=2
  Th : Inport  Port=3
  Divide2 : Product  Inputs=****/
  Subsystem : Subsystem
  d_h1 : Constant  Value=1.5
  lambda thermal conductivity of air [W/m/K] : Constant  Value=0.025
  QV_h_i : Outport
  wires:
  Divide2/1 -> QV_h_i/1
  Subsystem/2(dT) -> Divide2/4
  Subsystem/1(Gr) -> Divide2/2
  d_h1/1 -> Divide2/5
  A_h_exp/1 -> Divide2/3
  lambda thermal conductivity of air [W/m/K]/1 -> Divide2/1
  Th/1 -> Subsystem/2(Th)
  Ti/1 -> Subsystem/1(Ti)

== system MenakaModel/Control System/PID - constant setpoints - Ti measure/Subsystem1/Heating Controler/Subsystem/Subsystem2 ==
  Te : Inport
  A_h_exp : Inport  Port=2
  Th : Inport  Port=3
  Divide2 : Product  Inputs=****/
  Subsystem : Subsystem
  d_h1 : Constant  Value=1.5
  lambda thermal conductivity of air [W/m/K] : Constant  Value=0.025
  QV_h_e : Outport
  wires:
  Divide2/1 -> QV_h_e/1
  Subsystem/2(dT) -> Divide2/4
  Subsystem/1(Gr) -> Divide2/2
  d_h1/1 -> Divide2/5
  A_h_exp/1 -> Divide2/3
  lambda thermal conductivity of air [W/m/K]/1 -> Divide2/1
  Th/1 -> Subsystem/2(Th)
  Te/1 -> Subsystem/1(Ti)

== system MenakaModel/Control System/PID-set-points/Subsystem1/Heating Controler/Subsystem/Subsystem1 ==
  Ti : Inport
  A_h_exp : Inport  Port=2
  Th : Inport  Port=3
  Divide2 : Product  Inputs=****/
  Subsystem : Subsystem
  d_h1 : Constant  Value=1.5
  lambda thermal conductivity of air [W/m/K] : Constant  Value=0.025
  QV_h_i : Outport
  wires:
  Divide2/1 -> QV_h_i/1
  Subsystem/2(dT) -> Divide2/4
  Subsystem/1(Gr) -> Divide2/2
  d_h1/1 -> Divide2/5
  A_h_exp/1 -> Divide2/3
  lambda thermal conductivity of air [W/m/K]/1 -> Divide2/1
  Th/1 -> Subsystem/2(Th)
  Ti/1 -> Subsystem/1(Ti)

== system MenakaModel/Control System/PID-set-points/Subsystem1/Heating Controler/Subsystem/Subsystem2 ==
  Te : Inport
  A_h_exp : Inport  Port=2
  Th : Inport  Port=3
  Divide2 : Product  Inputs=****/
  Subsystem : Subsystem
  d_h1 : Constant  Value=1.5
  lambda thermal conductivity of air [W/m/K] : Constant  Value=0.025
  QV_h_e : Outport
  wires:
  Divide2/1 -> QV_h_e/1
  Subsystem/2(dT) -> Divide2/4
  Subsystem/1(Gr) -> Divide2/2
  d_h1/1 -> Divide2/5
  A_h_exp/1 -> Divide2/3
  lambda thermal conductivity of air [W/m/K]/1 -> Divide2/1
  Th/1 -> Subsystem/2(Th)
  Te/1 -> Subsystem/1(Ti)

== system MenakaModel/Control System/Setpoints Control - ON//OFF/Subsystem1/Heating Controler/Subsystem/Subsystem1 ==
  Ti : Inport
  A_h_exp : Inport  Port=2
  Th : Inport  Port=3
  Divide2 : Product  Inputs=****/
  Subsystem : Subsystem
  d_h1 : Constant  Value=1.5
  lambda thermal conductivity of air [W/m/K] : Constant  Value=0.025
  QV_h_i : Outport
  wires:
  Divide2/1 -> QV_h_i/1
  Subsystem/2(dT) -> Divide2/4
  Subsystem/1(Gr) -> Divide2/2
  d_h1/1 -> Divide2/5
  A_h_exp/1 -> Divide2/3
  lambda thermal conductivity of air [W/m/K]/1 -> Divide2/1
  Th/1 -> Subsystem/2(Th)
  Ti/1 -> Subsystem/1(Ti)

== system MenakaModel/Control System/Setpoints Control - ON//OFF/Subsystem1/Heating Controler/Subsystem/Subsystem2 ==
  Te : Inport
  A_h_exp : Inport  Port=2
  Th : Inport  Port=3
  Divide2 : Product  Inputs=****/
  Subsystem : Subsystem
  d_h1 : Constant  Value=1.5
  lambda thermal conductivity of air [W/m/K] : Constant  Value=0.025
  QV_h_e : Outport
  wires:
  Divide2/1 -> QV_h_e/1
  Subsystem/2(dT) -> Divide2/4
  Subsystem/1(Gr) -> Divide2/2
  d_h1/1 -> Divide2/5
  A_h_exp/1 -> Divide2/3
  lambda thermal conductivity of air [W/m/K]/1 -> Divide2/1
  Th/1 -> Subsystem/2(Th)
  Te/1 -> Subsystem/1(Ti)

== system MenakaModel/Control System/Control System Proportional (Ti) + Tmu Windows Relay/Windows Controler/Subsystem/Subsystem/Subsystem2/If Action Subsystem ==
  Action Port : ActionPort  ActionPortLabel=if(u2 > u1)
  Constant : Constant
  Out1 : Outport
  wires:
  Constant/1 -> Out1/1

== system MenakaModel/Control System/Control System Proportional (Ti) + Tmu Windows Relay/Windows Controler/Subsystem/Subsystem/Subsystem2/If Action Subsystem1 ==
  Action Port : ActionPort  ActionPortLabel=elseif(u2 < u3)
  Constant : Constant  Value=0
  Out1 : Outport
  wires:
  Constant/1 -> Out1/1

== system MenakaModel/Control System/Control System Proportional (Ti) + Tmu Windows Relay/Windows Controler/Subsystem/Subsystem/Subsystem2/If Action Subsystem2 ==
  In1 : Inport
  Action Port : ActionPort  ActionPortLabel=else
  Out1 : Outport
  wires:
  In1/1 -> Out1/1

== system MenakaModel/Control System/ON//OFF - constant setpoints/Subsystem1/Heating Controler/Subsystem/Subsystem1/Subsystem ==
  Ti : Inport
  Th : Inport  Port=2
  " nu kinematic viscosity [m^2/s]" : Constant  Value=15.1e-6
  Abs : Abs  SaturateOnIntegerOverflow=off
  Constant : Constant  Value=3
  Divide : Product  Inputs=*/
  Divide1 : Product  Inputs=*/
  Minus : Sum  Inputs=+-
  Power : Math  Operator=pow
  Product : Product
  Product1 : Product
  Square : Math  Operator=square
  d_h : Constant  Value=1.5
  g acceleration due to gravity [m/s^2] : Constant  Value=9.81
  Gr : Outport
  dT : Outport  Port=2
  wires:
  g acceleration due to gravity [m/s^2]/1 -> Product/1
  Abs/1 -> Divide/1
  Divide1/1 -> Product1/1
  Divide/1 -> Product1/2
  Product1/1 -> Gr/1
  Square/1 -> Divide1/2
  Product/1 -> Divide1/1
  Constant/1 -> Power/2
  Th/1 -> Minus/1
  " nu kinematic viscosity [m^2/s]"/1 -> Square/1
  Minus/1 -> dT/1, Abs/1
  d_h/1 -> Power/1
  Power/1 -> Product/2
  Ti/1 -> Divide/2, Minus/2

== system MenakaModel/Control System/ON//OFF - constant setpoints/Subsystem1/Heating Controler/Subsystem/Subsystem2/Subsystem ==
  Ti : Inport
  Th : Inport  Port=2
  " nu kinematic viscosity [m^2/s]" : Constant  Value=15.1e-6
  Abs : Abs  SaturateOnIntegerOverflow=off
  Constant : Constant  Value=3
  Divide : Product  Inputs=*/
  Divide1 : Product  Inputs=*/
  Minus : Sum  Inputs=+-
  Power : Math  Operator=pow
  Product : Product
  Product1 : Product
  Square : Math  Operator=square
  d_h : Constant  Value=1.5
  g acceleration due to gravity [m/s^2] : Constant  Value=9.81
  Gr : Outport
  dT : Outport  Port=2
  wires:
  g acceleration due to gravity [m/s^2]/1 -> Product/1
  Abs/1 -> Divide/1
  Divide1/1 -> Product1/1
  Divide/1 -> Product1/2
  Product1/1 -> Gr/1
  Square/1 -> Divide1/2
  Product/1 -> Divide1/1
  Constant/1 -> Power/2
  Th/1 -> Minus/1
  " nu kinematic viscosity [m^2/s]"/1 -> Square/1
  Minus/1 -> dT/1, Abs/1
  d_h/1 -> Power/1
  Power/1 -> Product/2
  Ti/1 -> Divide/2, Minus/2

== system MenakaModel/Control System/PID - const st - Ti mesure - Dynamics ST/Subsystem1/Heating Controler/Subsystem/Subsystem1/Subsystem ==
  Ti : Inport
  Th : Inport  Port=2
  " nu kinematic viscosity [m^2/s]" : Constant  Value=15.1e-6
  Abs : Abs  SaturateOnIntegerOverflow=off
  Constant : Constant  Value=3
  Divide : Product  Inputs=*/
  Divide1 : Product  Inputs=*/
  Minus : Sum  Inputs=+-
  Power : Math  Operator=pow
  Product : Product
  Product1 : Product
  Square : Math  Operator=square
  d_h : Constant  Value=1.5
  g acceleration due to gravity [m/s^2] : Constant  Value=9.81
  Gr : Outport
  dT : Outport  Port=2
  wires:
  g acceleration due to gravity [m/s^2]/1 -> Product/1
  Abs/1 -> Divide/1
  Divide1/1 -> Product1/1
  Divide/1 -> Product1/2
  Product1/1 -> Gr/1
  Square/1 -> Divide1/2
  Product/1 -> Divide1/1
  Constant/1 -> Power/2
  Th/1 -> Minus/1
  " nu kinematic viscosity [m^2/s]"/1 -> Square/1
  Minus/1 -> dT/1, Abs/1
  d_h/1 -> Power/1
  Power/1 -> Product/2
  Ti/1 -> Divide/2, Minus/2

== system MenakaModel/Control System/PID - const st - Ti mesure - Dynamics ST/Subsystem1/Heating Controler/Subsystem/Subsystem2/Subsystem ==
  Ti : Inport
  Th : Inport  Port=2
  " nu kinematic viscosity [m^2/s]" : Constant  Value=15.1e-6
  Abs : Abs  SaturateOnIntegerOverflow=off
  Constant : Constant  Value=3
  Divide : Product  Inputs=*/
  Divide1 : Product  Inputs=*/
  Minus : Sum  Inputs=+-
  Power : Math  Operator=pow
  Product : Product
  Product1 : Product
  Square : Math  Operator=square
  d_h : Constant  Value=1.5
  g acceleration due to gravity [m/s^2] : Constant  Value=9.81
  Gr : Outport
  dT : Outport  Port=2
  wires:
  g acceleration due to gravity [m/s^2]/1 -> Product/1
  Abs/1 -> Divide/1
  Divide1/1 -> Product1/1
  Divide/1 -> Product1/2
  Product1/1 -> Gr/1
  Square/1 -> Divide1/2
  Product/1 -> Divide1/1
  Constant/1 -> Power/2
  Th/1 -> Minus/1
  " nu kinematic viscosity [m^2/s]"/1 -> Square/1
  Minus/1 -> dT/1, Abs/1
  d_h/1 -> Power/1
  Power/1 -> Product/2
  Ti/1 -> Divide/2, Minus/2

== system MenakaModel/Control System/PID - constant setpoints/Subsystem1/Heating Controler/Subsystem/Subsystem1/Subsystem ==
  Ti : Inport
  Th : Inport  Port=2
  " nu kinematic viscosity [m^2/s]" : Constant  Value=15.1e-6
  Abs : Abs  SaturateOnIntegerOverflow=off
  Constant : Constant  Value=3
  Divide : Product  Inputs=*/
  Divide1 : Product  Inputs=*/
  Minus : Sum  Inputs=+-
  Power : Math  Operator=pow
  Product : Product
  Product1 : Product
  Square : Math  Operator=square
  d_h : Constant  Value=1.5
  g acceleration due to gravity [m/s^2] : Constant  Value=9.81
  Gr : Outport
  dT : Outport  Port=2
  wires:
  g acceleration due to gravity [m/s^2]/1 -> Product/1
  Abs/1 -> Divide/1
  Divide1/1 -> Product1/1
  Divide/1 -> Product1/2
  Product1/1 -> Gr/1
  Square/1 -> Divide1/2
  Product/1 -> Divide1/1
  Constant/1 -> Power/2
  Th/1 -> Minus/1
  " nu kinematic viscosity [m^2/s]"/1 -> Square/1
  Minus/1 -> dT/1, Abs/1
  d_h/1 -> Power/1
  Power/1 -> Product/2
  Ti/1 -> Divide/2, Minus/2

== system MenakaModel/Control System/PID - constant setpoints/Subsystem1/Heating Controler/Subsystem/Subsystem2/Subsystem ==
  Ti : Inport
  Th : Inport  Port=2
  " nu kinematic viscosity [m^2/s]" : Constant  Value=15.1e-6
  Abs : Abs  SaturateOnIntegerOverflow=off
  Constant : Constant  Value=3
  Divide : Product  Inputs=*/
  Divide1 : Product  Inputs=*/
  Minus : Sum  Inputs=+-
  Power : Math  Operator=pow
  Product : Product
  Product1 : Product
  Square : Math  Operator=square
  d_h : Constant  Value=1.5
  g acceleration due to gravity [m/s^2] : Constant  Value=9.81
  Gr : Outport
  dT : Outport  Port=2
  wires:
  g acceleration due to gravity [m/s^2]/1 -> Product/1
  Abs/1 -> Divide/1
  Divide1/1 -> Product1/1
  Divide/1 -> Product1/2
  Product1/1 -> Gr/1
  Square/1 -> Divide1/2
  Product/1 -> Divide1/1
  Constant/1 -> Power/2
  Th/1 -> Minus/1
  " nu kinematic viscosity [m^2/s]"/1 -> Square/1
  Minus/1 -> dT/1, Abs/1
  d_h/1 -> Power/1
  Power/1 -> Product/2
  Ti/1 -> Divide/2, Minus/2

== system MenakaModel/Control System/PID - constant setpoints - Ti measure/Subsystem1/Heating Controler/Subsystem/Subsystem1/Subsystem ==
  Ti : Inport
  Th : Inport  Port=2
  " nu kinematic viscosity [m^2/s]" : Constant  Value=15.1e-6
  Abs : Abs  SaturateOnIntegerOverflow=off
  Constant : Constant  Value=3
  Divide : Product  Inputs=*/
  Divide1 : Product  Inputs=*/
  Minus : Sum  Inputs=+-
  Power : Math  Operator=pow
  Product : Product
  Product1 : Product
  Square : Math  Operator=square
  d_h : Constant  Value=1.5
  g acceleration due to gravity [m/s^2] : Constant  Value=9.81
  Gr : Outport
  dT : Outport  Port=2
  wires:
  g acceleration due to gravity [m/s^2]/1 -> Product/1
  Abs/1 -> Divide/1
  Divide1/1 -> Product1/1
  Divide/1 -> Product1/2
  Product1/1 -> Gr/1
  Square/1 -> Divide1/2
  Product/1 -> Divide1/1
  Constant/1 -> Power/2
  Th/1 -> Minus/1
  " nu kinematic viscosity [m^2/s]"/1 -> Square/1
  Minus/1 -> dT/1, Abs/1
  d_h/1 -> Power/1
  Power/1 -> Product/2
  Ti/1 -> Divide/2, Minus/2

== system MenakaModel/Control System/PID - constant setpoints - Ti measure/Subsystem1/Heating Controler/Subsystem/Subsystem2/Subsystem ==
  Ti : Inport
  Th : Inport  Port=2
  " nu kinematic viscosity [m^2/s]" : Constant  Value=15.1e-6
  Abs : Abs  SaturateOnIntegerOverflow=off
  Constant : Constant  Value=3
  Divide : Product  Inputs=*/
  Divide1 : Product  Inputs=*/
  Minus : Sum  Inputs=+-
  Power : Math  Operator=pow
  Product : Product
  Product1 : Product
  Square : Math  Operator=square
  d_h : Constant  Value=1.5
  g acceleration due to gravity [m/s^2] : Constant  Value=9.81
  Gr : Outport
  dT : Outport  Port=2
  wires:
  g acceleration due to gravity [m/s^2]/1 -> Product/1
  Abs/1 -> Divide/1
  Divide1/1 -> Product1/1
  Divide/1 -> Product1/2
  Product1/1 -> Gr/1
  Square/1 -> Divide1/2
  Product/1 -> Divide1/1
  Constant/1 -> Power/2
  Th/1 -> Minus/1
  " nu kinematic viscosity [m^2/s]"/1 -> Square/1
  Minus/1 -> dT/1, Abs/1
  d_h/1 -> Power/1
  Power/1 -> Product/2
  Ti/1 -> Divide/2, Minus/2

== system MenakaModel/Control System/PID-set-points/Subsystem1/Heating Controler/Subsystem/Subsystem1/Subsystem ==
  Ti : Inport
  Th : Inport  Port=2
  " nu kinematic viscosity [m^2/s]" : Constant  Value=15.1e-6
  Abs : Abs  SaturateOnIntegerOverflow=off
  Constant : Constant  Value=3
  Divide : Product  Inputs=*/
  Divide1 : Product  Inputs=*/
  Minus : Sum  Inputs=+-
  Power : Math  Operator=pow
  Product : Product
  Product1 : Product
  Square : Math  Operator=square
  d_h : Constant  Value=1.5
  g acceleration due to gravity [m/s^2] : Constant  Value=9.81
  Gr : Outport
  dT : Outport  Port=2
  wires:
  g acceleration due to gravity [m/s^2]/1 -> Product/1
  Abs/1 -> Divide/1
  Divide1/1 -> Product1/1
  Divide/1 -> Product1/2
  Product1/1 -> Gr/1
  Square/1 -> Divide1/2
  Product/1 -> Divide1/1
  Constant/1 -> Power/2
  Th/1 -> Minus/1
  " nu kinematic viscosity [m^2/s]"/1 -> Square/1
  Minus/1 -> dT/1, Abs/1
  d_h/1 -> Power/1
  Power/1 -> Product/2
  Ti/1 -> Divide/2, Minus/2

== system MenakaModel/Control System/PID-set-points/Subsystem1/Heating Controler/Subsystem/Subsystem2/Subsystem ==
  Ti : Inport
  Th : Inport  Port=2
  " nu kinematic viscosity [m^2/s]" : Constant  Value=15.1e-6
  Abs : Abs  SaturateOnIntegerOverflow=off
  Constant : Constant  Value=3
  Divide : Product  Inputs=*/
  Divide1 : Product  Inputs=*/
  Minus : Sum  Inputs=+-
  Power : Math  Operator=pow
  Product : Product
  Product1 : Product
  Square : Math  Operator=square
  d_h : Constant  Value=1.5
  g acceleration due to gravity [m/s^2] : Constant  Value=9.81
  Gr : Outport
  dT : Outport  Port=2
  wires:
  g acceleration due to gravity [m/s^2]/1 -> Product/1
  Abs/1 -> Divide/1
  Divide1/1 -> Product1/1
  Divide/1 -> Product1/2
  Product1/1 -> Gr/1
  Square/1 -> Divide1/2
  Product/1 -> Divide1/1
  Constant/1 -> Power/2
  Th/1 -> Minus/1
  " nu kinematic viscosity [m^2/s]"/1 -> Square/1
  Minus/1 -> dT/1, Abs/1
  d_h/1 -> Power/1
  Power/1 -> Product/2
  Ti/1 -> Divide/2, Minus/2

== system MenakaModel/Control System/Setpoints Control - ON//OFF/Subsystem1/Heating Controler/Subsystem/Subsystem1/Subsystem ==
  Ti : Inport
  Th : Inport  Port=2
  " nu kinematic viscosity [m^2/s]" : Constant  Value=15.1e-6
  Abs : Abs  SaturateOnIntegerOverflow=off
  Constant : Constant  Value=3
  Divide : Product  Inputs=*/
  Divide1 : Product  Inputs=*/
  Minus : Sum  Inputs=+-
  Power : Math  Operator=pow
  Product : Product
  Product1 : Product
  Square : Math  Operator=square
  d_h : Constant  Value=1.5
  g acceleration due to gravity [m/s^2] : Constant  Value=9.81
  Gr : Outport
  dT : Outport  Port=2
  wires:
  g acceleration due to gravity [m/s^2]/1 -> Product/1
  Abs/1 -> Divide/1
  Divide1/1 -> Product1/1
  Divide/1 -> Product1/2
  Product1/1 -> Gr/1
  Square/1 -> Divide1/2
  Product/1 -> Divide1/1
  Constant/1 -> Power/2
  Th/1 -> Minus/1
  " nu kinematic viscosity [m^2/s]"/1 -> Square/1
  Minus/1 -> dT/1, Abs/1
  d_h/1 -> Power/1
  Power/1 -> Product/2
  Ti/1 -> Divide/2, Minus/2

== system MenakaModel/Control System/Setpoints Control - ON//OFF/Subsystem1/Heating Controler/Subsystem/Subsystem2/Subsystem ==
  Ti : Inport
  Th : Inport  Port=2
  " nu kinematic viscosity [m^2/s]" : Constant  Value=15.1e-6
  Abs : Abs  SaturateOnIntegerOverflow=off
  Constant : Constant  Value=3
  Divide : Product  Inputs=*/
  Divide1 : Product  Inputs=*/
  Minus : Sum  Inputs=+-
  Power : Math  Operator=pow
  Product : Product
  Product1 : Product
  Square : Math  Operator=square
  d_h : Constant  Value=1.5
  g acceleration due to gravity [m/s^2] : Constant  Value=9.81
  Gr : Outport
  dT : Outport  Port=2
  wires:
  g acceleration due to gravity [m/s^2]/1 -> Product/1
  Abs/1 -> Divide/1
  Divide1/1 -> Product1/1
  Divide/1 -> Product1/2
  Product1/1 -> Gr/1
  Square/1 -> Divide1/2
  Product/1 -> Divide1/1
  Constant/1 -> Power/2
  Th/1 -> Minus/1
  " nu kinematic viscosity [m^2/s]"/1 -> Square/1
  Minus/1 -> dT/1, Abs/1
  d_h/1 -> Power/1
  Power/1 -> Product/2
  Ti/1 -> Divide/2, Minus/2

== matlab function MenakaModel/Control System/ON//OFF - constant setpoints/Subsystem1/Windows Controler/Subsystem/Selection  ==
  data: Rad input; Temperature input; y output; Humidity input; Rad_threshold input
function y = fcn(Rad,Temperature,Humidity,Rad_threshold)

h = double(Rad > Rad_threshold);

y = h*Temperature + (1-h)*Humidity;

%y = Temperature;
